simulink model "SimulacionControlador1"  (R2023a)
settings: Solver=VariableStepAuto  StartTime=0.0  StopTime=5.0  RelTol=1e-3
libraries: simulink x2
settings Model: Creator=camil  LastModifiedBy=camil

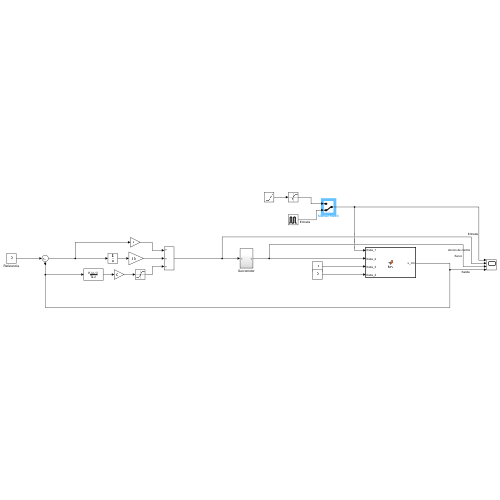
[thumbnail: Simulink's stored preview of the top-level diagram]
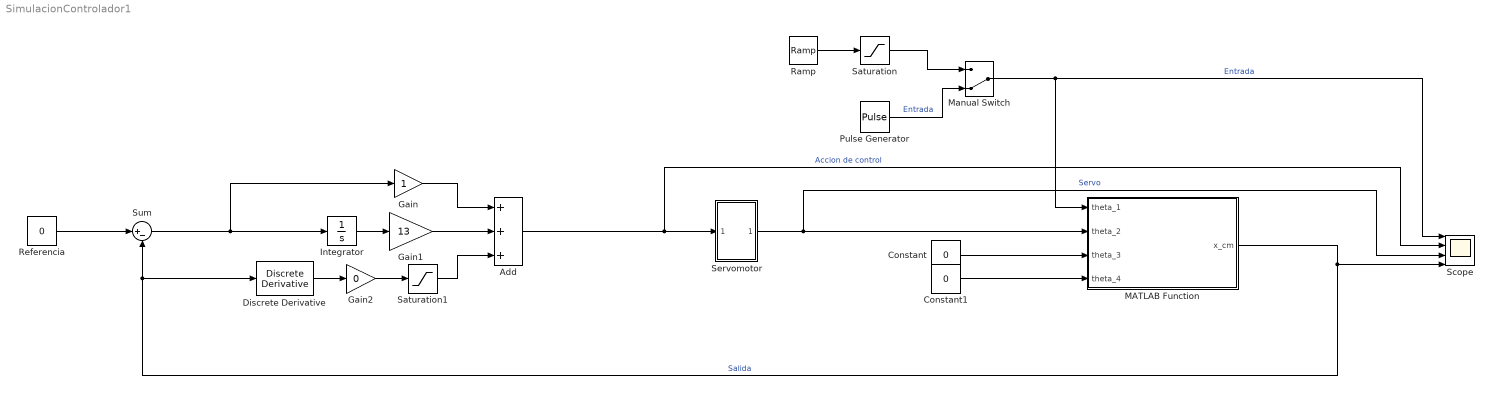
== system SimulacionControlador1 ==
  Add : Sum  Inputs=+++
  Constant : Constant  Value=0
  Constant1 : Constant  Value=0
  Discrete Derivative : simulink/Discrete/Discrete Derivative  gainval=1.0  ICPrevScaledInput=0.0  OutMin=[]  OutMax=[]  OutDataType=fixdt(1, 16)  OutScaling=2^-10  DoSatur=off
  Gain : Gain
  Gain1 : Gain  Gain=13
  Gain2 : Gain  Gain=0
  Integrator : Integrator
  MATLAB Function : MATLAB Function  TreatAsAtomicUnit=on
  Manual Switch : ManualSwitch  CurrentSetting=0
  Pulse Generator : DiscretePulseGenerator  PulseType=Time based  Amplitude=20  PulseWidth=50  PhaseDelay=1
  Ramp : simulink/Sources/Ramp  slope=10  start=1  InitialOutput=0
  Referencia : Constant  Value=0
  Saturation : Saturate  UpperLimit=10  LowerLimit=0
  Saturation1 : Saturate  UpperLimit=20  LowerLimit=-20
  Scope : Scope  NumInputPorts=4
  Servomotor : Subsystem
  Sum : Sum  Inputs=|+-
  wires:
  Referencia/1 -> Sum/1
  Gain/1 -> Add/1
  Gain1/1 -> Add/2
  Gain2/1 -> Saturation1/1
  Integrator/1 -> Gain1/1
  Discrete Derivative/1 -> Gain2/1
  MATLAB Function/1(x_cm) -> Discrete Derivative/1, Sum/2, Scope/4  "Salida"
  Sum/1 -> Integrator/1, Gain/1
  Constant/1 -> MATLAB Function/3(theta_3)
  Constant1/1 -> MATLAB Function/4(theta_4)
  Add/1 -> Scope/2, Servomotor/1(In1)  "Accion de control"
  Ramp/1 -> Saturation/1
  Servomotor/1(Out1) -> Scope/3, MATLAB Function/2(theta_2)  "Servo"
  Pulse Generator/1 -> Manual Switch/2  "Entrada"
  Saturation1/1 -> Add/3
  Manual Switch/1 -> Scope/1, MATLAB Function/1(theta_1)  "Entrada"
  Saturation/1 -> Manual Switch/1

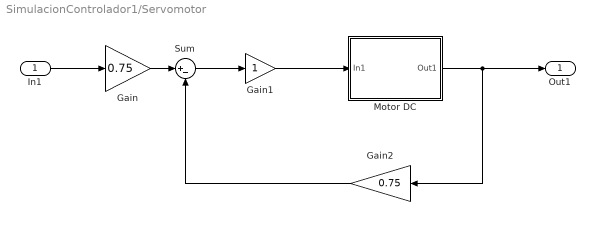
== system SimulacionControlador1/Servomotor ==
  In1 : Inport
  Gain : Gain  Gain=0.75
  Gain1 : Gain
  Gain2 : Gain  Gain=0.75
  Motor DC : Subsystem
  Sum : Sum  Inputs=|+-
  Out1 : Outport
  wires:
  Motor DC/1(Out1) -> Out1/1, Gain2/1
  Gain/1 -> Sum/1
  Sum/1 -> Gain1/1
  Gain2/1 -> Sum/2
  Gain1/1 -> Motor DC/1(In1)
  In1/1 -> Gain/1

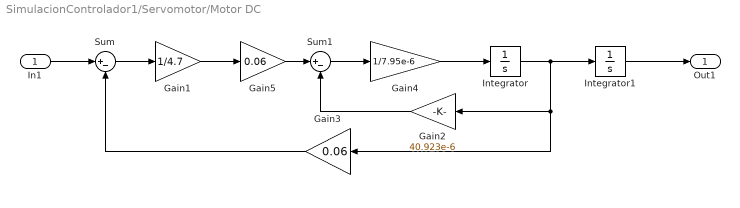
== system SimulacionControlador1/Servomotor/Motor DC ==
  In1 : Inport
  Gain1 : Gain  Gain=1/4.7
  Gain2 : Gain  Gain=40.923e-6
  Gain3 : Gain  Gain=0.06
  Gain4 : Gain  Gain=1/7.95e-6
  Gain5 : Gain  Gain=0.06
  Integrator : Integrator
  Integrator1 : Integrator
  Sum : Sum  Inputs=|+-
  Sum1 : Sum  Inputs=|+-
  Out1 : Outport
  wires:
  Gain2/1 -> Sum1/2
  Gain4/1 -> Integrator/1
  Sum1/1 -> Gain4/1
  Sum/1 -> Gain1/1
  Gain1/1 -> Gain5/1
  Gain3/1 -> Sum/2
  Integrator/1 -> Gain3/1, Gain2/1, Integrator1/1
  Gain5/1 -> Sum1/1
  In1/1 -> Sum/1
  Integrator1/1 -> Out1/1

== matlab function SimulacionControlador1/MATLAB Function ==
  data: theta_1 input; x_cm output; theta_2 input; theta_3 input; theta_4 input
function x_cm = fcn(theta_1, theta_2, theta_3, theta_4)

% Vector de posiciones angulares
theta = [theta_1, theta_2, theta_3, theta_4];

% Vector de longitudes
L = [4, 24.5, 29, 11];

% Vector de posiciones de articulaciones
x = [0, 0, 0, 0];

% Calculo de posiciones de articulaciones
theta_sum = 0;
x_ant = 0;
for i = 1:length(theta)
        
    %Posicion x anterior
    if i == 1
        x_ant = 0;
    else 
        x_ant = x(i-1);
    end
    
    %Sumatoria de angulos
    for j = 1:i
        theta_sum = theta_sum + theta(i);
    end
    
    x(i) = x_ant + L(i)*sin((pi*theta_sum)/180);
end

% Vector de pesos
weight = [500, 334, 500, 330];

% Centro de masa
x_cm = 0;

% Calculo centro de masa

M_t = sum(weight);
for i = 1:length(x)
    x_cm = x_cm + x(i)*weight(i);
end

x_cm = x_cm/M_t;
